simulink library "thc"  (R2021b)
settings: Solver=VariableStepAuto  StartTime=0.0  StopTime=10.0  RelTol=1e-3
undefined symbols (not defined in the file): ATHC_APTCQA_X_C, ATHC_APTCQB_X_C, ATHC_dAy_X_C, ATHC_Qeq_X_kmh, ATHC_VbaseC_X_C, ATHC_VbaseC_Y_W, ATHC_VbaseD_X_C, ATHC_VbaseH_X_C, FALSE, KTHC_ACMaxMinT_sec, KTHC_aDeice_K, KTHC_AGSDefLv_K, KTHC_AGSLv1_K, KTHC_AGSLv2_K, KTHC_AGSLv3_K, KTHC_AGSLv4_K, KTHC_AGSLv5_K, KTHC_AirIntUpdateT_sec, KTHC_APTCOneZoneMax_W, KTHC_APTCPeriod_cnt, KTHC_APTCPWMEN_flg, KTHC_APTCQMaxC_W, KTHC_APTCQminC_W, KTHC_APTCQminD_W, KTHC_APTCQminRe1_W, KTHC_APTCQminRe_W, KTHC_APTCQoffT_cnt, KTHC_APTCQonT_cnt, KTHC_APTCRiLeMaxDff_W, KTHC_APTCRiLeMinDff_W, KTHC_BatCoolT_cnt, KTHC_BatInTempDef_C, KTHC_bDeice_K, KTHC_CompMaxDeice_rpm, KTHC_CompMinDeice_rpm, KTHC_CompSotxvOp_K, KTHC_CompSotxvOpLow_rpm, KTHC_CompSpdmax_rpm, KTHC_CompSpdmaxBC1_rpm, KTHC_CompSpdmaxBC_rpm, KTHC_CompSpdmid1_rpm, KTHC_CompSpdmid2_rpm, KTHC_CompSpdmid3_rpm, KTHC_CompSpdmid_rpm, KTHC_CompSpdmin_rpm, KTHC_DAPTCQ1_W, KTHC_DAPTCQ2_W, KTHC_DAPTCQ3_W, KTHC_DcChSetTemp_C, KTHC_DehumidityEN_flg, KTHC_DeiceCycTime_K, KTHC_DriveLevelWPTCBAH1_W, KTHC_DriveLevelWPTCBAH2_W, KTHC_DriveLevelWPTCBAH3_W, KTHC_DriveLevelWPTCBAH4_W, KTHC_DriverSeatPos_flg, KTHC_DriveT1MinBAH_C, KTHC_DriveT2MaxBAH_C, KTHC_DriveT2MinBAH_C, KTHC_DriveT3MaxBAH_C ... (+379)
libraries: simulink x489
(part 15 of 17)

== stateflow chart thc/THC/ThermalControl/THCM_Conctrl/Chart1 ==
  state TambLevel
    state WaitForUpdate
    (default) -> (junction 43)
    WaitForUpdate -> (junction 43) [order 4] : [hasChanged(ECOSW)]
    (junction 43) -> (junction 19)
    WaitForUpdate -> (junction 19) [order 1] : [hasChanged(SetTempZon1St_CMD)]
    (junction 19) -> (junction 25)
    WaitForUpdate -> (junction 25) [order 2] : [hasChanged(SetTempZon2St_CMD)]
    (junction 25) -> (junction 21)
    WaitForUpdate -> (junction 21) [order 3] : [after(KTHC_ECOTambLVT_sec*10,tick)]
    (junction 21) -> (junction 46)
    (junction 46) -> WaitForUpdate [order 1] : [!ECOSW]{alpha=0;beta=0;sigSetTempZon1Stadj=sigSetTempZon1St;sigSetTempZon2Stadj=sigSetTempZon2St;}
    (junction 46) -> (junction 5) [order 2]
    (junction 5) -> (junction 29) [order 1] : [Tamb<KTHC_ECOTambLV1_C]{alpha=KTHC_ECOalpha1_K;beta=KTHC_ECObeta1_K;}
    (junction 5) -> (junction 7) [order 2]
    (junction 29) -> (junction 31)
    (junction 7) -> (junction 31) [order 1] : [Tamb<KTHC_ECOTambLV2_C]{alpha=KTHC_ECOalpha2_K;beta=KTHC_ECObeta2_K;}
    (junction 7) -> (junction 10) [order 2]
    (junction 31) -> (junction 34)
    (junction 10) -> (junction 34) [order 1] : [Tamb<KTHC_ECOTambLV3_C]{alpha=KTHC_ECOalpha3_K;beta=KTHC_ECObeta3_K;}
    (junction 10) -> (junction 13) [order 2]
    (junction 34) -> (junction 37)
    (junction 13) -> (junction 37) [order 1] : [Tamb<KTHC_ECOTambLV4_C]{alpha=KTHC_ECOalpha4_K;beta=KTHC_ECObeta4_K;}
    (junction 13) -> (junction 16) [order 2]
    (junction 37) -> (junction 40)
    (junction 16) -> (junction 40) [order 1] : [Tamb<KTHC_ECOTambLV5_C]{alpha=KTHC_ECOalpha5_K;beta=KTHC_ECObeta5_K;}
    (junction 16) -> (junction 110) [order 2]
    (junction 40) -> (junction 97)
    (junction 110) -> (junction 97) [order 1] : [Tamb<KTHC_ECOTambLV6_C]{alpha=KTHC_ECOalpha6_K;beta=KTHC_ECObeta6_K;}
    (junction 110) -> (junction 107) [order 2]
    (junction 97) -> (junction 95)
    (junction 107) -> (junction 95) [order 1] : [Tamb<KTHC_ECOTambLV7_C]{alpha=KTHC_ECOalpha7_K;beta=KTHC_ECObeta7_K;}
    (junction 107) -> (junction 103) [order 2]
    (junction 95) -> (junction 100)
    (junction 103) -> (junction 100) [order 1] : [Tamb<KTHC_ECOTambLV8_C]{alpha=KTHC_ECOalpha8_K;beta=KTHC_ECObeta8_K;}
    (junction 103) -> (junction 94) [order 2]
    (junction 100) -> (junction 102)
    (junction 94) -> (junction 102) : {alpha=KTHC_ECOalpha9_K;beta=KTHC_ECObeta9_K;}
    (junction 102) -> (junction 54) [order 1] : [sigSetTempZon1St<Tamb]
        | {sigSetTempZon1Stadj=sigSetTempZon1St-(sigSetTempZon1St-Tamb)*alpha;}
    (junction 102) -> (junction 55) [order 2]
    (junction 54) -> (junction 57)
    (junction 55) -> (junction 57) : {sigSetTempZon1Stadj=sigSetTempZon1St-(sigSetTempZon1St-Tamb)*beta;}
    (junction 57) -> WaitForUpdate [order 1] : [sigSetTempZon2St<Tamb]
        | {sigSetTempZon2Stadj=sigSetTempZon2St-(sigSetTempZon2St-Tamb)*alpha;}
    (junction 57) -> (junction 62) [order 2]
    (junction 62) -> WaitForUpdate : {sigSetTempZon2Stadj=sigSetTempZon2St-(sigSetTempZon2St-Tamb)*beta;}
  data: KTHC_ECOTambLV1_C input; KTHC_ECOTambLV2_C input; KTHC_ECOTambLV3_C input; KTHC_ECOTambLV4_C input; KTHC_ECOTambLV5_C input; KTHC_ECOTambLV6_C input; KTHC_ECOTambLV7_C input; KTHC_ECOTambLV8_C input; KTHC_ECOTambLVT_sec input; KTHC_ECOalpha1_K input; KTHC_ECOalpha2_K input; KTHC_ECOalpha3_K input; KTHC_ECOalpha4_K input; KTHC_ECOalpha5_K input; KTHC_ECOalpha6_K input; KTHC_ECOalpha7_K input; KTHC_ECOalpha8_K input; KTHC_ECObeta1_K input; KTHC_ECObeta2_K input; KTHC_ECObeta3_K input; KTHC_ECObeta4_K input; KTHC_ECObeta5_K input; KTHC_ECOalpha9_K input; KTHC_ECObeta6_K input; KTHC_ECObeta7_K input; KTHC_ECObeta8_K input; KTHC_ECObeta9_K input; Tamb input; sigSetTempZon1St input; SetTempZon1St_CMD input; sigSetTempZon1Stadj output double; alpha local double; beta local double; sigSetTempZon2St input; SetTempZon2St_CMD input; sigSetTempZon2Stadj output double; ECOSW input

== stateflow chart thc/THC/ThermalControl/THCM_Conctrl/CompCtrl/Enabled Subsystem1/Chart ==
  state Level1
    en:Bat_In_TempSetPoint=KTHC_T1winSetpointBC_C;
  state Level2
    en:Bat_In_TempSetPoint=KTHC_T2winSetpointBC_C;
  state Level3
    en:Bat_In_TempSetPoint=KTHC_T3winSetpointBC_C;
  state Level4
    en:Bat_In_TempSetPoint=KTHC_T4winSetpointBC_C;
  state Level5
    en:Bat_In_TempSetPoint=KTHC_T5winSetpointBC_C;
  (default) -> Level1
  Level1 -> Level2 : [TBMax>KTHC_T1MaxBC_C]
  Level2 -> Level1 [order 2] : [TBMax<KTHC_T2MinBC_C]
  Level2 -> Level3 [order 1] : [TBMax>KTHC_T2MaxBC_C]
  Level3 -> Level2 [order 2] : [TBMax<KTHC_T3MinBC_C]
  Level3 -> Level4 [order 1] : [TBMax>KTHC_T3MaxBC_C]
  Level4 -> Level3 [order 1] : [TBMax<KTHC_T4MinBC_C]
  Level4 -> Level5 [order 2] : [TBMax>KTHC_T4MaxBC_C]
  Level5 -> Level4 : [TBMax<KTHC_T5MinBC_C]
  data: TBMax input; Bat_In_TempSetPoint output; KTHC_T1MaxBC_C input; KTHC_T2MinBC_C input; KTHC_T2MaxBC_C input; KTHC_T3MinBC_C input; KTHC_T3MaxBC_C input; KTHC_T4MinBC_C input; KTHC_T4MaxBC_C input; KTHC_T5MinBC_C input; KTHC_T1winSetpointBC_C input; KTHC_T2winSetpointBC_C input; KTHC_T3winSetpointBC_C input; KTHC_T4winSetpointBC_C input; KTHC_T5winSetpointBC_C input

== stateflow chart thc/THC/ThermalControl/THCM_Conctrl/APTC/Chart1 ==
  state OFF
    en:APTCset=0;
  state ONOFF
    state ON
      en:APTCset=KTHC_APTCQminC_W;
    state OFF
      en:APTCset=0;
    (default) -> ON
    ON -> ONOFF.OFF : [after(KTHC_APTCQonT_cnt,tick)]
    ONOFF.OFF -> ON : [after(KTHC_APTCQoffT_cnt,tick)]
  (default) -> OFF
  OFF -> ONOFF : [APTCPID==8]
  ONOFF -> OFF : [APTCPID!=8]
  data: KTHC_APTCQminC_W input; APTCPID input; KTHC_APTCQonT_cnt input; KTHC_APTCQoffT_cnt input; APTCset output double
